simulink model "motorbb_ideal"  (R2023a)
settings: Solver=VariableStepAuto  StartTime=0.0  StopTime=15  RelTol=1e-3
undefined symbols (not defined in the file or in its folder): ke0, p0
settings Model: Creator=Matlab  LastModifiedBy=erwinplanck
settings ModelReferenceCC: EnableRefExpFcnMdlSchedulingChecks=on

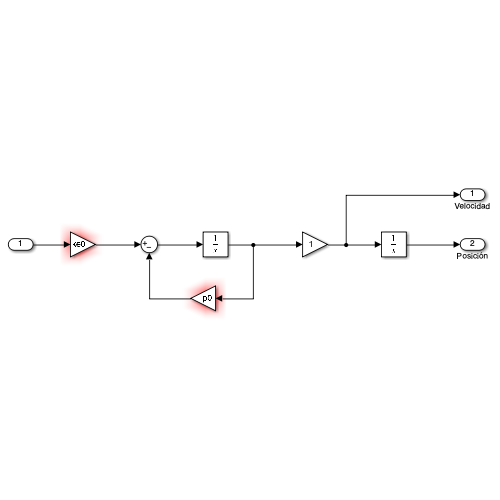
[thumbnail: Simulink's stored preview of the top-level diagram]
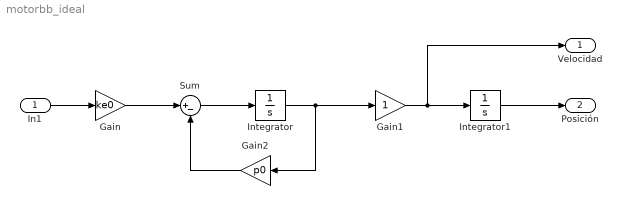
== system motorbb_ideal ==
  In1 : Inport
  Gain : Gain  Gain=ke0
  Gain1 : Gain
  Gain2 : Gain  Gain=p0
  Integrator : Integrator
  Integrator1 : Integrator
  Sum : Sum  Inputs=|+-
  Velocidad : Outport
  Posición : Outport  Port=2
  wires:
  In1/1 -> Gain/1
  Gain/1 -> Sum/1
  Sum/1 -> Integrator/1
  Integrator/1 -> Gain2/1, Gain1/1
  Gain1/1 -> Velocidad/1, Integrator1/1
  Gain2/1 -> Sum/2
  Integrator1/1 -> Posición/1
